simulink model "temp_onoff_ctrl"  (Simulink 7.4)
settings: Solver=ode4  StartTime=0.0  StopTime=1800  FixedStep=1  RelTol=1e-3
CloseFcn:
  | rtwprivate ssgencode ModelCloseRequest adc1
settings Model: Creator=BMTD  LastModifiedBy=BMTD  SimulationMode=external  ExtModeEnableFloating=off  ExtModeTrigDuration=100000  ExtModeArchiveMode=auto  ExtModeArchiveFileName=vd1  ExtModeArchiveDirName=B:\temp
settings DataIOCC: LimitDataPoints=off  SaveOutput=off  SignalLogging=off  SaveTime=off
settings OptimizationCC: InitFltsAndDblsToZero=on
settings DebuggingCC: SaveWithParameterizedLinksMsg=none  SignalResolutionControl=TryResolveAllWithWarning  MultiTaskDSMMsg=warning  MultiTaskCondExecSysMsg=none  StrictBusMsg=ErrorLevel1
settings RTWCC: SystemTargetFile=rtwin.tlc  TemplateMakefile=rtwin.tmf  Description=Real-Time Windows Target  ProcessScript=rtwin_make_rtw_hook  IncludeERTFirstTime=on
settings RTWCC: CustomSourceCode=|
  | /* list of Real-Time Windows Target boards */
  | const int RTWinBoardCount = 4;
  | RTWINBOARD RTWinBoards[4] = {
  |   { "Standard_Devices/Generic_8-bit_Port", LPT_CTRL, 0, NULL },
  |   { "Standard_Devices/Generic_8-bit_Port", LPT_ADDR, 0, NULL },
  |   { "Standard_Devices/Generic_8-bit_Port", LPT_DATA, 0, NULL },
  |   { "Standard_Devices/Generic_8-bit_Port", LPT_ECPR, 0, NULL },
  | };
  | 
  | int32_T Channels = 0;
  | int32_T BitMode = 1;
  | 
  | 
  | 
  | /*
  |  * Ham doc muc logic tu port DIN o J6
  |  * Gia tri tra ve 8bit tuong ung DI7-DI0
  |  * address: dia chi giai ma
  |  */
  | real_T inport (real_T address)
  | {
  |     real_T addrval, dataval;
  | 	int i;
  | 
  |     addrval = address;
  | 
  |     RTBIO_DriverIO(EPP_ADDR, DIGITALOUTPUT, IOWRITE, 1, &Channels, &addrval, &BitMode);
  | 	for(i=0; i<1000; i++);
  |     RTBIO_DriverIO(EPP_DATA, DIGITALINPUT, IOREAD, 1, &Channels, &dataval, &BitMode);
  | 	for(i=0; i<1000; i++);
  | 
  |     return  dataval;
  | }
  | 
  | 
  | /*
  |  * Ham xuat muc logic ra port DOUT o J8
  |  * data: gia tri 8bit tuong ung DO7-DO0
  |  * address: dia chi giai ma
  |  */
  | void outport (real_T address, real_T data)
  | {
  |     real_T addrval, dataval;
  | 	int i;
  | 
  |     addrval = address;
  |     dataval = data;
  | 
  |     RTBIO_DriverIO(EPP_ADDR, DIGITALOUTPUT, IOWRITE, 1, &Channels, &addrval, &BitMode);
  | 	for(i=0; i<1000; i++);
  |     RTBIO_DriverIO(EPP_DATA, DIGITALOUTPUT, IOWRITE, 1, &Channels, &dataval, &BitMode);
  |     for(i=0; i<1000; i++);
  | }
  | 
  | 
  | /*
  |  * Ham reset 4 kenh encoder o J5
  |  * Sau khi reset gia tri encoder tro ve 1.000.000
  |  * channel: 1-4 tuong ung voi ENC_CH1 - ENC_CH4
  |  */
  | void encoder_reset (real_T channel)
  | {
  | 	real_T temp;
  | 
  | 	temp = pow(2.0,(channel-1.0));
  | 
  | 	outport(ENC_RESET, temp);
  | 	outport(ENC_RESET, 16.0);
  | }
  | 
  | /*
  |  * Ham chot du lieu 4 kenh encoder o J5
  |  * Sau khi chot gia tri encoder duoc du nguyen
  |  * channel: 1-4 tuong ung voi ENC_CH1 - ENC_CH4
  |  */
  | void encoder_latch (real_T channel)
  | {
  | 	real_T temp;
  | 
  | 	temp = pow(2.0,(channel-1.0));
  | 
  | 	outport(ENC_LATCH, temp);
  | 	outport(ENC_LATCH, 16.0);
  | }
  | 
  | /*
  |  * Ham doc 4 kenh encoder o J5
  |  * Gia tri tra ve 21bit
  |  * channel: 1-4 tuong ung voi ENC_CH1 - ENC_CH4
  |  */
  | real_T encoder_read (real_T channel)
  | {
  | 	real_T  d, d1, d2, d3, temp;
  | 
  | 	encoder_latch(channel);
  | 
  | 	temp = ENC_CH1 + 3.0*(channel-1.0);
  | 	d1 = inport(temp);
  | 	d2 = inport(temp + 1.0);
  | 	d3 = inport(temp + 2.0);
  | 
  | 	d = d3*65536.0 + d2*256.0 + d1;
  | 
  | 	return d;
  | }
  | 
  | 
  | /*
  |  * Ham doc 4 kenh toc do tu encoder o J5
  |  * Gia tri tra ve 16bit: (B15:B0) don vi 0.2us
  |  * Voi Encoder 400xung, toc do 3000rpm, do rong 1 xung la 50us
  |  * Toc do (rpm) = 750.000 / (B14:B0)
  |  * B15 = 1 neu quay thuan, = 0 neu quay nghich
  |  * channel: 1-4 tuong ung voi SPD_CH1 - SPD_CH4
  |  */
  | real_T speed_read (real_T channel)
  | {
  | 	real_T  d, d1, d2, temp;
  | 
  | 	temp = SPD_CH1 + 2.0*(channel-1.0);
  | 	d1 = inport(temp);
  | 	d2 = inport(temp + 1.0);
  | 
  | 	d = d2*256.0 + d1;
  | 
  |     if ((d==32000.0)||(d==64768.0))
  |         d = 1000000.0; //xem nhu toc do = 0
  | 	else if (d >32768.0)    d = d-32768.0;
  | 	else   d = -d;
  | 
  | 	return d;
  | }
  | 
  | 
  | /*
  |  * Ham cho phep ngo ra dieu rong xung
  |  */
  | void pwm_enable (void)
  | {
  | 	outport(PWM_ENA, 15.0);
  | }
  | 
  | 
  | /*
  |  * Ham cam ngo ra dieu rong xung
  |  */
  | void pwm_disable (void)
  | {
  | 	outport(PWM_ENA, 16.0);
  | }
  | 
  | 
  | 
  | /*
  |  * Ham cai dat khoang thoi gian dieu rong xung
  |  * T: 1-50 <don vi 0.1ms>
  |  */
  | void pwm_set_T (real_T T)
  | {
  | 
  | 	real_T temp;
  | 
  | 	temp = T;
  | 
  | 	if(temp <= 1.0)  temp = 1.0;
  | 	else  temp = 2*temp - 1.0;
  | 
  | 	if(temp >100.0)  temp = 100.0;
  | 
  | 	outport(PWM_FDIV, temp);
  | 
  | }
  | 
  | 
  | /*
  |  * Ham cai dat khoang thoi gian dieu rong xung
  |  * T: 1-50 <don vi 0.1s>
  |  */
  | void pwm_set_Ts (real_T T)
  | {
  | 	real_T temp;
  | 
  | 	temp = T;
  | 
  | 	if(temp <= 1.0)  temp = 1.0;
  | 	else  temp = 2*temp - 1.0;
  | 
  | 	if(temp >100.0)  temp = 100.0;
  | 
  |     temp = temp + 127.0;  // giam 1 de Matlab xuat dung (dung la 128.0)
  | 	outport(PWM_FDIV, temp);
  | 
  | }
  | 
  | 
  | /*
  |  * Ham nap gia tri do rong xung vao 4 kenh pwm
  |  * channel: 1-4 tuong ung voi 4 motor
  |  * Ton: -1000 den 1000 tuong ung voi -100.0% den 100.0% <do phan giai 0.1%>
  |  */
  | void pwm_write (real_T channel, real_T Ton)
  | {
  | 	real_T dh, dl, d;
  | 	real_T dir, temp;
  | 
  | 	temp = Ton;
  | 	dir  = 0.0;
  | 
  | 	if (temp < 0.0){
  | 		temp = -temp;
  | 		dir  = 1.0;
  | 	}
  |     if (temp >800.0) temp = 800.0;   // han che toc do o 80%
  | 
  | 	temp = dir*1024.0 + temp;
  | 	dh = floor(temp/256.0);
  | 	dl = (temp/256.0 - dh)*256.0;
  | 
  | 	if (dl == 0.0)   dl = 0.1;
  | 	if (dh == 0.0)   dh = 16.0;
  | 
  | 	outport(PWM_DATAL, dl);
  | 	outport(PWM_DATAH, dh);
  | 
  | 	d = pow(2.0, (channel-1.0));	// lua chon kenh pwm
  | 	outport(PWM_CTRL, d);			// tao xung canh len
  | 	outport(PWM_CTRL, 16.0);		// de nap vao fifo
  | }
  | 
  | 
  | /*
  |  * Ham doc gia tri ADC cua cac kenh
  |  * channel: 1-3 tuong ung voi 3 kenh ADC
  |  * Gia tri tra ve 12bit ADC
  |  */
  | real_T adc_read (real_T channel)
  | {
  | 	real_T temp;
  | 	real_T d, d1, d2;
  | 
  | 	temp = ADC_CH1 + 2.0*(channel-1.0);
  | 
  | 	d1 = inport(temp);
  | 	d2 = inport(temp + 1.0);
  | 	d  = (d2*256.0 + d1);
  | 
  | 	return d;
  | }
  | 
  | 
  | /*
  |  * Ham xuat gia tri DAC ra cac kenh analog
  |  * channel: 1-3 tuong ung voi 3 kenh DAC
  |  * value: 0 - 4095
  |  */
  | void dac_write (real_T channel, real_T value)
  | {
  | 	real_T temp, dl, dh;
  | 
  | 	// lua chon kenh ket hop voi gia tri can xuat
  | 	temp = value;
  | 	if (temp <=0.0)  temp = 1.0;		// them vao 1 de Matlab xuat dung
  | 	else if (temp >4095.0)  temp = 4095.0;
  | 
  | 	temp = 4096.0*(channel - 1.0) + temp;
  | 
  | 	dh = floor(temp/256.0);
  | 	dl = (temp/256.0 - dh)*256.0;
  | 
  | 	// xuat gia tri DA ra kenh analog
  | 	outport(DAC_DOL, dl);
  | 	outport(DAC_DOH, dh);
  | 
  | 	outport(DAC_CTR, 1.0);	// tao xung canh len
  | 	outport(DAC_CTR, 16.0);	// de viet toi SPI
  | 
  | }
  | 
  | 
  | /* Ham khoi tao cong printer port o EPP mode
  |  * va reset cac ngoai vi
  |  */
  | void board_init(void)
  | {
  | 	real_T dataval1, dataval2;
  | 
  | 	// config EPP mode from cmos ECP mode
  | 	dataval1 = (double)0x80;
  | 	RTBIO_DriverIO(EPP_ECPR, DIGITALOUTPUT, IOWRITE, 1, &Channels, &dataval1, &BitMode);
  | 
  | 	// initialize EPP mode
  | 	dataval2 = (double)0x04;
  | 	RTBIO_DriverIO(EPP_CTRL, DIGITALOUTPUT, IOWRITE, 1, &Channels, &dataval2, &BitMode);
  | }
settings RTWCC: CustomHeaderCode=|
  | // printer port registers definition
  | #define     LPT_BASE    888U
  | #define     LPT_CTRL    890U
  | #define     LPT_ADDR    891U
  | #define     LPT_DATA    892U
  | #define     LPT_ECPR    1914U
  | 
  | #define     EPP_CTRL    0U
  | #define     EPP_ADDR    1U
  | #define     EPP_DATA    2U
  | #define     EPP_ECPR    3U
  | 
  | 
  | // IO module: Digital Input (1) and Digital Output (1)
  | #define		IO_IN		0x60		// J6
  | #define		IO_OUT		0x61		// J8
  | 
  | // ENCODER module (4)
  | #define		ENC_CH1		0x10		// J5
  | #define		ENC_CH2		0x13		// J5
  | #define		ENC_CH3		0x16		// J5
  | #define		ENC_CH4		0x19		// J5
  | #define		ENC_RESET	0x1C
  | #define		ENC_LATCH	0x1E
  | 
  | // SPEED module (4)
  | #define		SPD_CH1		0x20		// J5
  | #define		SPD_CH2		0x22		// J5
  | #define		SPD_CH3		0x24		// J5
  | #define		SPD_CH4		0x26		// J5
  | 
  | // ADC module: 3 analog inputs
  | #define		ADC_CH1		0x30		// J9
  | #define		ADC_CH2		0x32		// J9
  | #define		ADC_CH3		0x34		// J9
  | 
  | // DAC module: 3 analog outputs
  | #define		DAC_DOL		0x40		// J10
  | #define		DAC_DOH		0x41		// J10
  | #define		DAC_CTR		0x42		// J10
  | 
  | // PWM module
  | #define		PWM_DATAL	0x50		// J7
  | #define		PWM_DATAH	0x51		// J7
  | #define		PWM_FDIV	0x52		// J7
  | #define		PWM_CTRL	0x53		// J7
  | #define		PWM_ENA		0x54		// J7
  | 
  | 
  | 
  | // functions
  | real_T inport (real_T address);
  | void outport (real_T address, real_T data);
  | 
  | void encoder_reset (real_T channel);
  | void encoder_latch (real_T channel);
  | real_T encoder_read (real_T channel);
  | real_T speed_read (real_T channel);
  | 
  | void pwm_enable (void);
  | void pwm_disable (void);
  | void pwm_set_T (real_T T);
  | void pwm_set_Ts (real_T T);
  | void pwm_write (real_T channel, real_T Ton);
  | 
  | real_T adc_read (real_T channel);
  | void dac_write (real_T channel, real_T value);
  | 
  | void board_init(void);
settings RTWinTargetCC: TargetFcnLib=ansi_tfl_tmw.mat  TargetLibSuffix=_rtwin.lib  TargetPreCompLibLocation=C:\MATLABR2009b\toolbox\rtw\targets\rtwin\lib  TargetFunctionLibrary=ANSI_C  ModelReferenceCompliant=off  CompOptLevelCompliant=off  PortableWordSizes=off

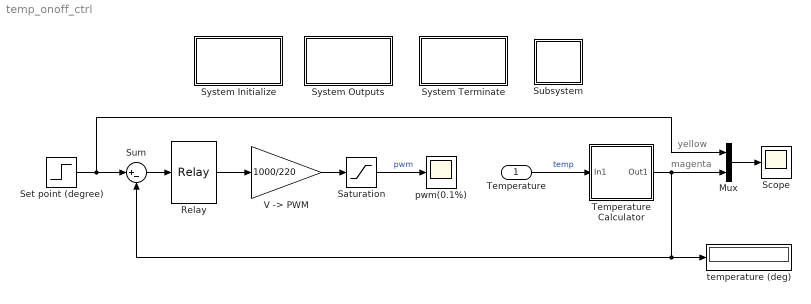
== system temp_onoff_ctrl ==
  note: yellow
  note: magenta
  Temperature : Inport  OutDataType=sfix(16)  OutScaling=2^0
  Mux : Mux  Inputs=2
  Relay : Relay  OnSwitchValue=1  OffSwitchValue=-1  OnOutputValue=1000  OutDataType=sfix(16)  OutScaling=2^0
  Saturation : Saturate  UpperLimit=800  LowerLimit=0.1
  Scope : Scope
      settings: YMin=0  YMax=130
  Set point (degree) : Step  Time=0  After=100  SampleTime=0
  Subsystem : Subsystem  TreatAsAtomicUnit=on
  Sum : Sum  Inputs=|+-  OutDataType=sfix(16)  OutScaling=2^0
  System Initialize : Subsystem  mask(System Initialize){ShowInLibBrowser=0}
      mask prompts: ShowInLibBrowser "Mask Parameter 1:"
      mask help: Add code to a systems Initialize function
      settings: CopyFcn=cccopyfcn(gcb)  OpenFcn=ccopenfcn('System Initialize Function')
      mask Help: This block contains text fields to insert custom user code sections at the declaration, execution and exit sections of the systems initialize function.  By placing this block inside a subsytem, the custom user code will appear in that subsystems function.
      mask Display: disp('System\nInitialize');
  System Outputs : Subsystem  mask(System Outputs){ShowInLibBrowser=0}
      mask prompts: ShowInLibBrowser "Mask Parameter 1:"
      mask help: Add code to a systems Outputs function
      settings: CopyFcn=cccopyfcn(gcb)  OpenFcn=ccopenfcn('System Outputs Function')
      mask Help: This block contains text fields to insert custom user code sections at the declaration, execution and exit sections of the systems outputs function.  By placing this block inside a subsytem, the custom user code will appear in that subsystems function.
      mask Display: disp('System\nOutputs');
  System Terminate : Subsystem  mask(System Terminate){ShowInLibBrowser=0}
      mask prompts: ShowInLibBrowser "Mask Parameter 1:"
      mask help: Add code to a systems Terminate function
      settings: CopyFcn=cccopyfcn(gcb)  OpenFcn=ccopenfcn('System Terminate Function')
      mask Help: This block contains text fields to insert custom user code sections at the declaration, execution and exit sections of the systems terminate function.  By placing this block inside a subsytem, the custom user code will appear in that subsystems function.
      mask Display: disp('System\nTerminate');
  Temperature Calculator : Subsystem
  "V -> PWM" : Gain  Gain=1000/220  ParameterDataType=sfix(16)  ParameterScaling=2^0  OutDataType=sfix(16)  OutScaling=2^0  ParamDataTypeStr=Inherit: Same as input
  pwm(0.1%) : Scope
      settings: YMin=0  YMax=1000  DataFormat=Array
  temperature (deg) : Display
  wires:
  Sum/1 -> Relay/1
  Set point (degree)/1 -> Sum/1, Mux/1
  Mux/1 -> Scope/1
  Saturation/1 -> pwm(0.1%)/1  "pwm"
  Temperature Calculator/1(Out1) -> Mux/2, Sum/2, temperature (deg)/1
  Temperature/1 -> Temperature Calculator/1(In1)  "temp"
  "V -> PWM"/1 -> Saturation/1
  Relay/1 -> "V -> PWM"/1

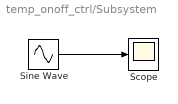
== system temp_onoff_ctrl/Subsystem ==
  Scope : Scope
  Sine Wave : Sin  Amplitude=1  Bias=0  Frequency=1  Phase=0  Samples=10  SampleTime=0  Offset=0
  wires:
  Sine Wave/1 -> Scope/1

== system temp_onoff_ctrl/System Initialize ==

== system temp_onoff_ctrl/System Outputs ==

== system temp_onoff_ctrl/System Terminate ==

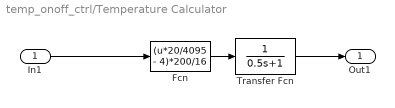
== system temp_onoff_ctrl/Temperature Calculator ==
  In1 : Inport  OutDataType=sfix(16)  OutScaling=2^0
  Fcn : Fcn  Expr=(u*20/4095 - 4)*200/16
  Transfer Fcn : TransferFcn  Denominator=[0.5 1]
  Out1 : Outport  OutDataType=sfix(16)  OutScaling=2^0
  wires:
  Transfer Fcn/1 -> Out1/1
  In1/1 -> Fcn/1
  Fcn/1 -> Transfer Fcn/1
